simulink model "attitude_model"  (R2019a)
settings: Solver=FixedStepAuto  StartTime=0.0  StopTime=100  FixedStep=0.01  RelTol=1e-3
settings Model: Creator=Duong  LastModifiedBy=Duong

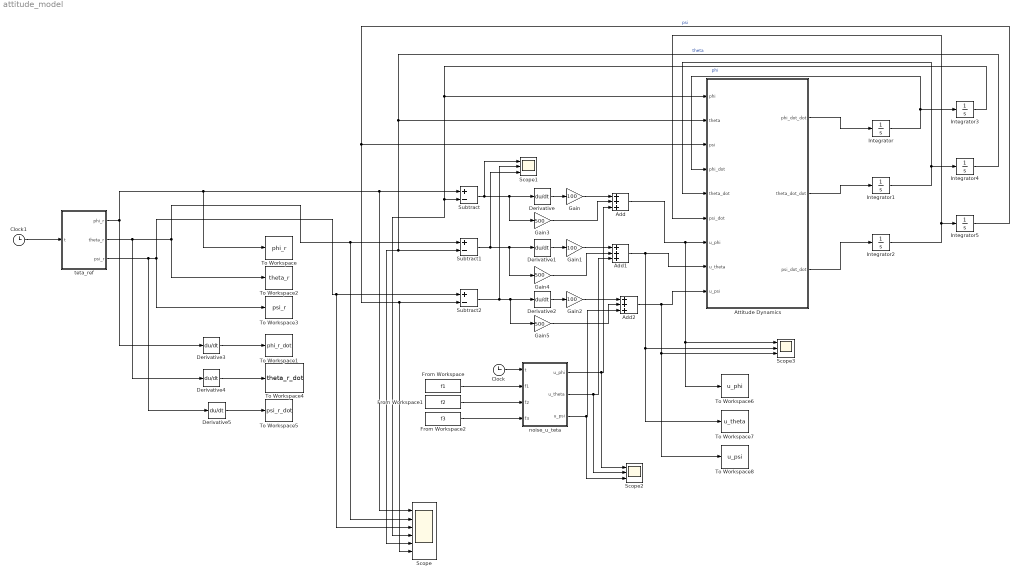
== system attitude_model ==
  Add : Sum  Inputs=+++
  Add1 : Sum  Inputs=+++
  Add2 : Sum  Inputs=+++
  Attitude Dynamics : MATLAB Function  TreatAsAtomicUnit=on
  Clock : Clock
  Clock1 : Clock
  Derivative{,1..5} (6 alike) : Derivative
  From Workspace : FromWorkspace  VariableName=f1  SampleTime=0
  From Workspace1 : FromWorkspace  VariableName=f2  SampleTime=0
  From Workspace2 : FromWorkspace  VariableName=f3  SampleTime=0
  Gain : Gain  Gain=100
  Gain1 : Gain  Gain=100
  Gain2 : Gain  Gain=100
  Gain3 : Gain  Gain=500
  Gain4 : Gain  Gain=500
  Gain5 : Gain  Gain=500
  Integrator : Integrator
  Integrator1 : Integrator
  Integrator2 : Integrator
  Integrator3 : Integrator  InitialCondition=0.5
  Integrator4 : Integrator  InitialCondition=0.8
  Integrator5 : Integrator  InitialCondition=-0.1
  Scope : Scope  NumInputPorts=6
  Scope1 : Scope  NumInputPorts=3
  Scope2 : Scope  NumInputPorts=3
  Scope3 : Scope  NumInputPorts=3
  Subtract : Sum  Inputs=+-
  Subtract1 : Sum  Inputs=+-
  Subtract2 : Sum  Inputs=+-
  To Workspace : ToWorkspace  VariableName=phi_r  SampleTime=-1
      settings: Save2DSignal=2-D array (concatenate along first dimension)
  To Workspace1 : ToWorkspace  VariableName=phi_r_dot  SampleTime=-1
      settings: Save2DSignal=2-D array (concatenate along first dimension)
  To Workspace2 : ToWorkspace  VariableName=theta_r  SampleTime=-1
      settings: Save2DSignal=2-D array (concatenate along first dimension)
  To Workspace3 : ToWorkspace  VariableName=psi_r  SampleTime=-1
      settings: Save2DSignal=2-D array (concatenate along first dimension)
  To Workspace4 : ToWorkspace  VariableName=theta_r_dot  SampleTime=-1
      settings: Save2DSignal=2-D array (concatenate along first dimension)
  To Workspace5 : ToWorkspace  VariableName=psi_r_dot  SampleTime=-1
      settings: Save2DSignal=2-D array (concatenate along first dimension)
  To Workspace6 : ToWorkspace  VariableName=u_phi  SampleTime=-1
      settings: Save2DSignal=2-D array (concatenate along first dimension)
  To Workspace7 : ToWorkspace  VariableName=u_theta  SampleTime=-1
      settings: Save2DSignal=2-D array (concatenate along first dimension)
  To Workspace8 : ToWorkspace  VariableName=u_psi  SampleTime=-1
      settings: Save2DSignal=2-D array (concatenate along first dimension)
  noise_u_teta : MATLAB Function  TreatAsAtomicUnit=on
  teta_ref : MATLAB Function  TreatAsAtomicUnit=on
  wires:
  Attitude Dynamics/1(phi_dot_dot) -> Integrator/1
  Integrator/1 -> Attitude Dynamics/4(phi_dot), Integrator3/1
  Attitude Dynamics/2(theta_dot_dot) -> Integrator1/1
  Integrator1/1 -> Attitude Dynamics/5(theta_dot), Integrator4/1
  Attitude Dynamics/3(psi_dot_dot) -> Integrator2/1
  Integrator2/1 -> Attitude Dynamics/6(psi_dot), Integrator5/1
  Integrator3/1 -> Scope/4, Subtract/2, Attitude Dynamics/1(phi)  "phi"
  Integrator4/1 -> Subtract1/2, Scope/5, Attitude Dynamics/2(theta)  "theta"
  Integrator5/1 -> Subtract2/2, Scope/6, Attitude Dynamics/3(psi)  "psi"
  Derivative/1 -> Gain/1
  Subtract/1 -> Gain3/1, Derivative/1, Scope1/1
  Subtract1/1 -> Scope1/3, Gain4/1, Derivative1/1
  Derivative1/1 -> Gain1/1
  Subtract2/1 -> Scope1/2, Gain5/1, Derivative2/1
  Derivative2/1 -> Gain2/1
  Gain/1 -> Add/1
  Gain3/1 -> Add/2
  Gain1/1 -> Add1/1
  Gain4/1 -> Add1/2
  Gain2/1 -> Add2/1
  Gain5/1 -> Add2/2
  Add/1 -> Scope3/1, To Workspace6/1, Attitude Dynamics/7(u_phi)
  Add1/1 -> To Workspace7/1, Scope3/2, Attitude Dynamics/8(u_theta)
  Add2/1 -> To Workspace8/1, Scope3/3, Attitude Dynamics/9(u_psi)
  Clock/1 -> noise_u_teta/1(t)
  noise_u_teta/1(u_phi) -> Scope2/1, Add/3
  noise_u_teta/2(u_theta) -> Scope2/2, Add1/3
  noise_u_teta/3(u_psi) -> Scope2/3, Add2/3
  Derivative3/1 -> To Workspace1/1
  Clock1/1 -> teta_ref/1(t)
  teta_ref/1(phi_r) -> Derivative3/1, To Workspace/1, Scope/1, Subtract/1
  teta_ref/2(theta_r) -> Derivative4/1, To Workspace2/1, Scope/2, Subtract1/1
  teta_ref/3(psi_r) -> Derivative5/1, To Workspace3/1, Scope/3, Subtract2/1
  Derivative4/1 -> To Workspace4/1
  Derivative5/1 -> To Workspace5/1
  From Workspace/1 -> noise_u_teta/2(f1)
  From Workspace1/1 -> noise_u_teta/3(f2)
  From Workspace2/1 -> noise_u_teta/4(f3)

== matlab function attitude_model/noise_u_teta ==
  data: t input; u_phi output; u_theta output; u_psi output; f1 input; f2 input; f3 input
function [u_phi,u_theta,u_psi] = fcn(t,f1,f2,f3)
a=1; 
%global f1 f2 f3;
if(t<0  )
u_phi = sum(a*sin(f1*t));
u_theta = sum(a*sin(f2*t));
u_psi = sum(a*sin(f3*t));

else 
    
u_phi=0;
u_theta=0;
u_psi=0;
% omega_m = [1 2 3 5 6 7 8 11 13 15];
% e = [sum(0.01*sin(omega_m*t))]*ones(3,1);
% u0 = zeros(3,1);
% u  = u0 + e;
% u_phi=u(1);
% u_theta=u(2);
% u_psi=u(3);
% u_phi = sum(a*sin([1 3 7 11 13 15]*t));
% u_theta = sum(a*sin([1 3 7 11 13 15]*t));
% u_psi = sum(a*sin([1 3 7 11 13 15]*t));
end

== matlab function attitude_model/Attitude Dynamics ==
  data: phi input; theta input; phi_dot_dot output; theta_dot_dot output; psi_dot_dot output; psi input; phi_dot input; theta_dot input; psi_dot input; u_phi input; u_theta input; u_psi input
function [phi_dot_dot, theta_dot_dot, psi_dot_dot] = fcn(phi,theta,psi,phi_dot,theta_dot,psi_dot,u_phi,u_theta,u_psi)

teta_dot_dot=[0;0;0];
phi_dot_dot=0; theta_dot_dot=0; psi_dot_dot=0;
m=2.0;
J=diag([5.1,5.1,10.2]);
k_w=1;
k_t=1;
g=9.8;
l_to=0.2;
J_theta=5.1; J_phi=5.1; J_psi=10.2;
u_teta=[u_phi;u_theta;u_psi];
R=[cos(theta)*cos(psi) (cos(psi)*sin(phi)*sin(theta)-cos(phi)*sin(psi)) (sin(phi)*sin(psi)+cos(phi)*cos(psi)*sin(theta));
    cos(theta)*sin(psi) (cos(phi)*cos(psi)+sin(phi)*sin(theta)*sin(psi)) (cos(phi)*sin(theta)*sin(psi)-cos(psi)*sin(phi));
-sin(theta) (cos(theta)*sin(phi)) (cos(phi)*cos(theta))];


c11=0;
c12=(J_theta-J_psi)*(theta_dot*cos(phi)*sin(phi)+psi_dot*sin(phi)^2*cos(theta))/J_phi+((J_psi-J_theta)*psi_dot*cos(phi)^2*cos(theta)-J_phi*psi_dot*cos(theta))/J_phi;
c13=(J_psi-J_theta)*psi_dot*cos(phi)*sin(phi)*cos(theta)^2/J_phi;
c21=(J_psi-J_theta)*(theta_dot*cos(phi)*sin(phi)+psi_dot*sin(phi)^2*cos(theta))/J_theta+((J_theta-J_psi)*psi_dot*cos(phi)^2*cos(theta)+J_phi*psi_dot*cos(theta))/J_theta;
c22=(J_psi-J_theta)*phi_dot*cos(phi)*sin(phi)/J_theta;
c23=(-J_phi*psi_dot*sin(theta)*cos(theta)+J_psi*psi_dot*cos(phi)^2*cos(theta)*sin(theta))/J_theta+psi_dot*sin(phi)^2*cos(theta)*sin(theta);
c31=((J_theta-J_psi)*psi_dot*cos(theta)^2*sin(phi)*cos(phi)-J_phi*theta_dot*cos(theta))/J_psi;
c32=(J_psi-J_theta)*(theta_dot*cos(phi)*sin(phi)*sin(theta)+phi_dot*sin(phi)^2*cos(theta))/J_psi+((J_theta-J_psi)*phi_dot*cos(phi)^2*cos(theta)+J_phi*psi_dot*sin(theta)*cos(theta))/J_psi-J_theta*psi_dot*sin(phi)^2*sin(theta)*cos(theta)/J_psi-psi_dot*cos(phi)^2*cos(theta)*sin(theta);
c33=(-J_psi*theta_dot*cos(phi)^2*sin(theta)*cos(theta)-J_theta*theta_dot*sin(phi)^2*cos(theta)*sin(theta))/J_psi+((J_theta-J_psi)*phi_dot*cos(phi)*sin(phi)*cos(theta)^2+J_phi*theta_dot*sin(theta)*cos(theta))/J_psi;
C=[c11 c12 c13;
    c21 c22 c23;
    c31 c32 c33];
teta_dot=[phi_dot;theta_dot;psi_dot];
B=inv(J)*diag([(l_to*k_w),(l_to*k_w),(k_t)]);

teta_dot_dot=-inv(J)*C*teta_dot+B*u_teta;
phi_dot_dot=teta_dot_dot(1);
theta_dot_dot=teta_dot_dot(2);
psi_dot_dot=teta_dot_dot(3);

== matlab function attitude_model/teta_ref ==
  data: t input; phi_r output; theta_r output; psi_r output
function [phi_r, theta_r, psi_r] = fcn(t)
a=0.8;
f=0.1;
phi_r=a*sin(2*pi*f*t);
theta_r=a*sin(2*pi*f*t+pi/2);
psi_r=a*sin(2*pi*f*t+1);
phi_r=0;
theta_r=0;
psi_r=0;

a=0.9;
f=0.1;
phi_r=a*sin(2*pi*f*t)*exp(-0.8*t);
theta_r=a*cos(2*pi*f*t)*exp(-0.8*t);
psi_r=a*sin(2*pi*f*t+1)*exp(-0.8*t);
% phi_r=a*sin(2*pi*f*t);
% theta_r=a*cos(2*pi*f*t);
% psi_r=a*cos(2*pi*f*t+1);
psi_r=0;
